simulink model "untitled"  (R2019a)
settings: Solver=VariableStepAuto  StartTime=0.0  StopTime=10.0  RelTol=1e-3
values from neighbouring files (symbols this model uses):
  Jt = J'    [inverseDyn-test.m]
  KI = double(K_I(1))    [PD.m]    (also in inverseDyn-test.m = 1)
  KP = double(K_P(1))    [PD.m]    (also in inverseDyn-test.m = 1)
settings Model: Creator=JanAriel  LastModifiedBy=JanAriel

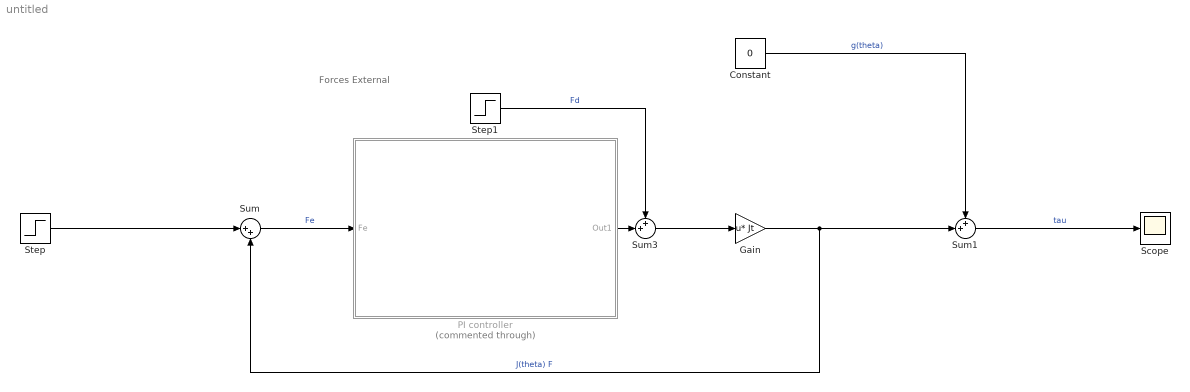
== system untitled ==
  note: Forces External
  Constant : Constant  Value=0
  Gain : Gain  Gain=Jt  Multiplication=Matrix(u*K)
  PI controller : Subsystem  Commented=through
  Scope : Scope
  Step : Step  Before=[0;0]  After=[25;25]  SampleTime=0
  Step1 : Step  SampleTime=0
  Sum : Sum  Inputs=|++
  Sum1 : Sum  Inputs=++|
  Sum3 : Sum  Inputs=++|
  wires:
  Constant/1 -> Sum1/1  "g(theta)"
  Gain/1 -> Sum1/2, Sum/2  "J(theta) F"
  Step/1 -> Sum/1
  Sum3/1 -> Gain/1
  Step1/1 -> Sum3/1  "Fd"
  Sum1/1 -> Scope/1  "tau"
  Sum/1 -> PI controller/1(Fe)  "Fe"
  PI controller/1(Out1) -> Sum3/2

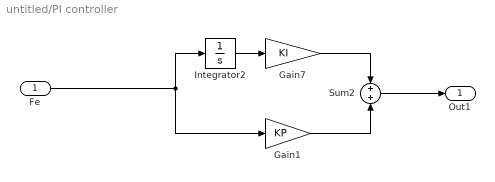
== system untitled/PI controller ==
  Fe : Inport
  Gain1 : Gain  Gain=KP
  Gain7 : Gain  Gain=KI
  Integrator2 : Integrator
  Sum2 : Sum
  Out1 : Outport
  wires:
  Integrator2/1 -> Gain7/1
  Gain1/1 -> Sum2/2
  Gain7/1 -> Sum2/1
  Sum2/1 -> Out1/1
  Fe/1 -> Gain1/1, Integrator2/1
